simulink model "MIMO_FixedIO"  (R2024a)
settings: Solver=VariableStepAuto  StartTime=0.0  StopTime=10  RelTol=1e-3
undefined symbols (not defined in the file or in its folder): BOOL, DINT, slplc
(part 2 of 5)

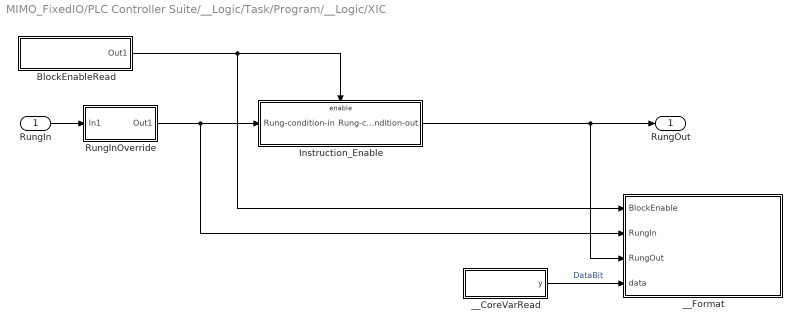
== system MIMO_FixedIO/PLC Controller Suite/__Logic/Task/Program/__Logic/XIC ==
  RungIn : Inport  PortDimensions=1
  BlockEnableRead : Subsystem  DisableCoverage=on  TreatAsAtomicUnit=on  mask{PLCLabelTag=_Block_Enable, PLCBlockType=BlockEnableRead}
      mask prompts: PLCLabelTag "Label Tag:"
      mask init:
      | block = gcb;
      | maskObj = Simulink.Mask.get(block);
      | maskObj.Display = sprintf('disp(''%s'');', PLCLabelTag);
      mask Help: web([docroot '/plccoder/ref/blockenableread' '.html']);
      mask DialogControl PLCBlockTitle Prompt: Block Enable Read
      mask Display: disp('_Block_Enable');
  Instruction_Enable : Subsystem  Priority=12  TreatAsAtomicUnit=on
  RungInOverride : Subsystem  DisableCoverage=on  TreatAsAtomicUnit=on
  __CoreVarRead : Subsystem  Tag=CoreVarReadBlock  DisableCoverage=on  TreatAsAtomicUnit=on  mask{PLCBlockType=CoreVarRead}
      mask init:
      | slplc.callbacks.initCoreVariable(gcb, 'read');
      mask Help: web([docroot '/plccoder/ref/__corevarread' '.html']);
      mask DialogControl PLCBlockTitle Prompt: Core Variable Read
  __Format : MATLAB Function  Tag=PLC_Format_Boolean  Priority=20  DisableCoverage=on  InitFcn=slplc.utils.setBlockAppearance('reset', '%<PLCOperandTag>');  StopFcn=slplc.utils.setBlockAppearance('reset', '%<PLCOperandTag>');  TreatAsAtomicUnit=on
  RungOut : Outport  OutDataTypeStr=BOOL  PortDimensions=1  InitialOutput=false  VectorParamsAs1DForOutWhenUnconnected=off
  wires:
  __CoreVarRead/1(y) -> __Format/4(data)  "DataBit"
  RungInOverride/1(Out1) -> Instruction_Enable/1(Rung-condition-in), __Format/2(RungIn)
  BlockEnableRead/1(Out1) -> Instruction_Enable/Enable, __Format/1(BlockEnable)
  Instruction_Enable/1(Rung-condition-out) -> RungOut/1, __Format/3(RungOut)
  RungIn/1 -> RungInOverride/1(In1)

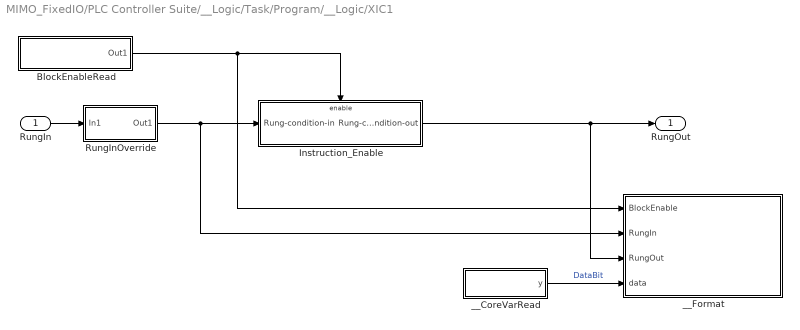
== system MIMO_FixedIO/PLC Controller Suite/__Logic/Task/Program/__Logic/XIC1 ==
  RungIn : Inport  PortDimensions=1
  BlockEnableRead : Subsystem  DisableCoverage=on  TreatAsAtomicUnit=on  mask{PLCLabelTag=_Block_Enable, PLCBlockType=BlockEnableRead}
      mask prompts: PLCLabelTag "Label Tag:"
      mask init:
      | block = gcb;
      | maskObj = Simulink.Mask.get(block);
      | maskObj.Display = sprintf('disp(''%s'');', PLCLabelTag);
      mask Help: web([docroot '/plccoder/ref/blockenableread' '.html']);
      mask DialogControl PLCBlockTitle Prompt: Block Enable Read
      mask Display: disp('_Block_Enable');
  Instruction_Enable : Subsystem  Priority=12  TreatAsAtomicUnit=on
  RungInOverride : Subsystem  DisableCoverage=on  TreatAsAtomicUnit=on
  __CoreVarRead : Subsystem  Tag=CoreVarReadBlock  DisableCoverage=on  TreatAsAtomicUnit=on  mask{PLCBlockType=CoreVarRead}
      mask init:
      | slplc.callbacks.initCoreVariable(gcb, 'read');
      mask Help: web([docroot '/plccoder/ref/__corevarread' '.html']);
      mask DialogControl PLCBlockTitle Prompt: Core Variable Read
  __Format : MATLAB Function  Tag=PLC_Format_Boolean  Priority=20  DisableCoverage=on  InitFcn=slplc.utils.setBlockAppearance('reset', '%<PLCOperandTag>');  StopFcn=slplc.utils.setBlockAppearance('reset', '%<PLCOperandTag>');  TreatAsAtomicUnit=on
  RungOut : Outport  OutDataTypeStr=BOOL  PortDimensions=1  InitialOutput=false  VectorParamsAs1DForOutWhenUnconnected=off
  wires:
  __CoreVarRead/1(y) -> __Format/4(data)  "DataBit"
  RungInOverride/1(Out1) -> Instruction_Enable/1(Rung-condition-in), __Format/2(RungIn)
  BlockEnableRead/1(Out1) -> Instruction_Enable/Enable, __Format/1(BlockEnable)
  Instruction_Enable/1(Rung-condition-out) -> RungOut/1, __Format/3(RungOut)
  RungIn/1 -> RungInOverride/1(In1)

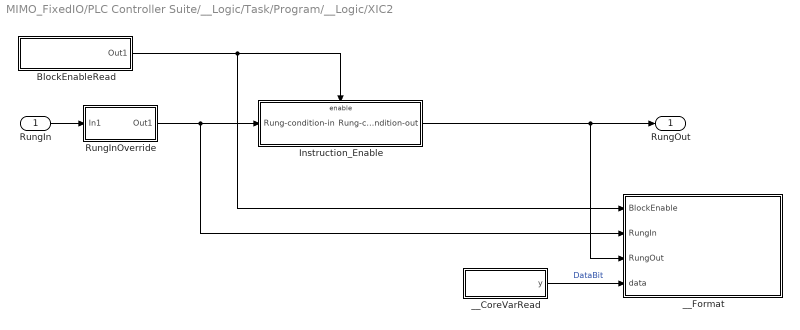
== system MIMO_FixedIO/PLC Controller Suite/__Logic/Task/Program/__Logic/XIC2 ==
  RungIn : Inport  PortDimensions=1
  BlockEnableRead : Subsystem  DisableCoverage=on  TreatAsAtomicUnit=on  mask{PLCLabelTag=_Block_Enable, PLCBlockType=BlockEnableRead}
      mask prompts: PLCLabelTag "Label Tag:"
      mask init:
      | block = gcb;
      | maskObj = Simulink.Mask.get(block);
      | maskObj.Display = sprintf('disp(''%s'');', PLCLabelTag);
      mask Help: web([docroot '/plccoder/ref/blockenableread' '.html']);
      mask DialogControl PLCBlockTitle Prompt: Block Enable Read
      mask Display: disp('_Block_Enable');
  Instruction_Enable : Subsystem  Priority=12  TreatAsAtomicUnit=on
  RungInOverride : Subsystem  DisableCoverage=on  TreatAsAtomicUnit=on
  __CoreVarRead : Subsystem  Tag=CoreVarReadBlock  DisableCoverage=on  TreatAsAtomicUnit=on  mask{PLCBlockType=CoreVarRead}
      mask init:
      | slplc.callbacks.initCoreVariable(gcb, 'read');
      mask Help: web([docroot '/plccoder/ref/__corevarread' '.html']);
      mask DialogControl PLCBlockTitle Prompt: Core Variable Read
  __Format : MATLAB Function  Tag=PLC_Format_Boolean  Priority=20  DisableCoverage=on  InitFcn=slplc.utils.setBlockAppearance('reset', '%<PLCOperandTag>');  StopFcn=slplc.utils.setBlockAppearance('reset', '%<PLCOperandTag>');  TreatAsAtomicUnit=on
  RungOut : Outport  OutDataTypeStr=BOOL  PortDimensions=1  InitialOutput=false  VectorParamsAs1DForOutWhenUnconnected=off
  wires:
  __CoreVarRead/1(y) -> __Format/4(data)  "DataBit"
  RungInOverride/1(Out1) -> Instruction_Enable/1(Rung-condition-in), __Format/2(RungIn)
  BlockEnableRead/1(Out1) -> Instruction_Enable/Enable, __Format/1(BlockEnable)
  Instruction_Enable/1(Rung-condition-out) -> RungOut/1, __Format/3(RungOut)
  RungIn/1 -> RungInOverride/1(In1)

== system MIMO_FixedIO/PLC Controller Suite/__Logic/Task/Program/__Logic/XIC3 ==
  RungIn : Inport  PortDimensions=1
  BlockEnableRead : Subsystem  DisableCoverage=on  TreatAsAtomicUnit=on  mask{PLCLabelTag=_Block_Enable, PLCBlockType=BlockEnableRead}
      mask prompts: PLCLabelTag "Label Tag:"
      mask init:
      | block = gcb;
      | maskObj = Simulink.Mask.get(block);
      | maskObj.Display = sprintf('disp(''%s'');', PLCLabelTag);
      mask Help: web([docroot '/plccoder/ref/blockenableread' '.html']);
      mask DialogControl PLCBlockTitle Prompt: Block Enable Read
      mask Display: disp('_Block_Enable');
  Instruction_Enable : Subsystem  Priority=12  TreatAsAtomicUnit=on
  RungInOverride : Subsystem  DisableCoverage=on  TreatAsAtomicUnit=on
  __CoreVarRead : Subsystem  Tag=CoreVarReadBlock  DisableCoverage=on  TreatAsAtomicUnit=on  mask{PLCBlockType=CoreVarRead}
      mask init:
      | slplc.callbacks.initCoreVariable(gcb, 'read');
      mask Help: web([docroot '/plccoder/ref/__corevarread' '.html']);
      mask DialogControl PLCBlockTitle Prompt: Core Variable Read
  __Format : MATLAB Function  Tag=PLC_Format_Boolean  Priority=20  DisableCoverage=on  InitFcn=slplc.utils.setBlockAppearance('reset', '%<PLCOperandTag>');  StopFcn=slplc.utils.setBlockAppearance('reset', '%<PLCOperandTag>');  TreatAsAtomicUnit=on
  RungOut : Outport  OutDataTypeStr=BOOL  PortDimensions=1  InitialOutput=false  VectorParamsAs1DForOutWhenUnconnected=off
  wires:
  __CoreVarRead/1(y) -> __Format/4(data)  "DataBit"
  RungInOverride/1(Out1) -> Instruction_Enable/1(Rung-condition-in), __Format/2(RungIn)
  BlockEnableRead/1(Out1) -> Instruction_Enable/Enable, __Format/1(BlockEnable)
  Instruction_Enable/1(Rung-condition-out) -> RungOut/1, __Format/3(RungOut)
  RungIn/1 -> RungInOverride/1(In1)

== system MIMO_FixedIO/PLC Controller Suite/__Logic/Task/Program/__Logic/XIC4 ==
  RungIn : Inport  PortDimensions=1
  BlockEnableRead : Subsystem  DisableCoverage=on  TreatAsAtomicUnit=on  mask{PLCLabelTag=_Block_Enable, PLCBlockType=BlockEnableRead}
      mask prompts: PLCLabelTag "Label Tag:"
      mask init:
      | block = gcb;
      | maskObj = Simulink.Mask.get(block);
      | maskObj.Display = sprintf('disp(''%s'');', PLCLabelTag);
      mask Help: web([docroot '/plccoder/ref/blockenableread' '.html']);
      mask DialogControl PLCBlockTitle Prompt: Block Enable Read
      mask Display: disp('_Block_Enable');
  Instruction_Enable : Subsystem  Priority=12  TreatAsAtomicUnit=on
  RungInOverride : Subsystem  DisableCoverage=on  TreatAsAtomicUnit=on
  __CoreVarRead : Subsystem  Tag=CoreVarReadBlock  DisableCoverage=on  TreatAsAtomicUnit=on  mask{PLCBlockType=CoreVarRead}
      mask init:
      | slplc.callbacks.initCoreVariable(gcb, 'read');
      mask Help: web([docroot '/plccoder/ref/__corevarread' '.html']);
      mask DialogControl PLCBlockTitle Prompt: Core Variable Read
  __Format : MATLAB Function  Tag=PLC_Format_Boolean  Priority=20  DisableCoverage=on  InitFcn=slplc.utils.setBlockAppearance('reset', '%<PLCOperandTag>');  StopFcn=slplc.utils.setBlockAppearance('reset', '%<PLCOperandTag>');  TreatAsAtomicUnit=on
  RungOut : Outport  OutDataTypeStr=BOOL  PortDimensions=1  InitialOutput=false  VectorParamsAs1DForOutWhenUnconnected=off
  wires:
  __CoreVarRead/1(y) -> __Format/4(data)  "DataBit"
  RungInOverride/1(Out1) -> Instruction_Enable/1(Rung-condition-in), __Format/2(RungIn)
  BlockEnableRead/1(Out1) -> Instruction_Enable/Enable, __Format/1(BlockEnable)
  Instruction_Enable/1(Rung-condition-out) -> RungOut/1, __Format/3(RungOut)
  RungIn/1 -> RungInOverride/1(In1)

== system MIMO_FixedIO/PLC Controller Suite/__Logic/Task/Program/__Logic/XIC5 ==
  RungIn : Inport  PortDimensions=1
  BlockEnableRead : Subsystem  DisableCoverage=on  TreatAsAtomicUnit=on  mask{PLCLabelTag=_Block_Enable, PLCBlockType=BlockEnableRead}
      mask prompts: PLCLabelTag "Label Tag:"
      mask init:
      | block = gcb;
      | maskObj = Simulink.Mask.get(block);
      | maskObj.Display = sprintf('disp(''%s'');', PLCLabelTag);
      mask Help: web([docroot '/plccoder/ref/blockenableread' '.html']);
      mask DialogControl PLCBlockTitle Prompt: Block Enable Read
      mask Display: disp('_Block_Enable');
  Instruction_Enable : Subsystem  Priority=12  TreatAsAtomicUnit=on
  RungInOverride : Subsystem  DisableCoverage=on  TreatAsAtomicUnit=on
  __CoreVarRead : Subsystem  Tag=CoreVarReadBlock  DisableCoverage=on  TreatAsAtomicUnit=on  mask{PLCBlockType=CoreVarRead}
      mask init:
      | slplc.callbacks.initCoreVariable(gcb, 'read');
      mask Help: web([docroot '/plccoder/ref/__corevarread' '.html']);
      mask DialogControl PLCBlockTitle Prompt: Core Variable Read
  __Format : MATLAB Function  Tag=PLC_Format_Boolean  Priority=20  DisableCoverage=on  InitFcn=slplc.utils.setBlockAppearance('reset', '%<PLCOperandTag>');  StopFcn=slplc.utils.setBlockAppearance('reset', '%<PLCOperandTag>');  TreatAsAtomicUnit=on
  RungOut : Outport  OutDataTypeStr=BOOL  PortDimensions=1  InitialOutput=false  VectorParamsAs1DForOutWhenUnconnected=off
  wires:
  __CoreVarRead/1(y) -> __Format/4(data)  "DataBit"
  RungInOverride/1(Out1) -> Instruction_Enable/1(Rung-condition-in), __Format/2(RungIn)
  BlockEnableRead/1(Out1) -> Instruction_Enable/Enable, __Format/1(BlockEnable)
  Instruction_Enable/1(Rung-condition-out) -> RungOut/1, __Format/3(RungOut)
  RungIn/1 -> RungInOverride/1(In1)

== system MIMO_FixedIO/PLC Controller Suite/__Logic/Task/Program/__Logic/XIC6 ==
  RungIn : Inport  PortDimensions=1
  BlockEnableRead : Subsystem  DisableCoverage=on  TreatAsAtomicUnit=on  mask{PLCLabelTag=_Block_Enable, PLCBlockType=BlockEnableRead}
      mask prompts: PLCLabelTag "Label Tag:"
      mask init:
      | block = gcb;
      | maskObj = Simulink.Mask.get(block);
      | maskObj.Display = sprintf('disp(''%s'');', PLCLabelTag);
      mask Help: web([docroot '/plccoder/ref/blockenableread' '.html']);
      mask DialogControl PLCBlockTitle Prompt: Block Enable Read
      mask Display: disp('_Block_Enable');
  Instruction_Enable : Subsystem  Priority=12  TreatAsAtomicUnit=on
  RungInOverride : Subsystem  DisableCoverage=on  TreatAsAtomicUnit=on
  __CoreVarRead : Subsystem  Tag=CoreVarReadBlock  DisableCoverage=on  TreatAsAtomicUnit=on  mask{PLCBlockType=CoreVarRead}
      mask init:
      | slplc.callbacks.initCoreVariable(gcb, 'read');
      mask Help: web([docroot '/plccoder/ref/__corevarread' '.html']);
      mask DialogControl PLCBlockTitle Prompt: Core Variable Read
  __Format : MATLAB Function  Tag=PLC_Format_Boolean  Priority=20  DisableCoverage=on  InitFcn=slplc.utils.setBlockAppearance('reset', '%<PLCOperandTag>');  StopFcn=slplc.utils.setBlockAppearance('reset', '%<PLCOperandTag>');  TreatAsAtomicUnit=on
  RungOut : Outport  OutDataTypeStr=BOOL  PortDimensions=1  InitialOutput=false  VectorParamsAs1DForOutWhenUnconnected=off
  wires:
  __CoreVarRead/1(y) -> __Format/4(data)  "DataBit"
  RungInOverride/1(Out1) -> Instruction_Enable/1(Rung-condition-in), __Format/2(RungIn)
  BlockEnableRead/1(Out1) -> Instruction_Enable/Enable, __Format/1(BlockEnable)
  Instruction_Enable/1(Rung-condition-out) -> RungOut/1, __Format/3(RungOut)
  RungIn/1 -> RungInOverride/1(In1)

== system MIMO_FixedIO/PLC Controller Suite/__Logic/Task/Program/__Logic/XIC8 ==
  RungIn : Inport  PortDimensions=1
  BlockEnableRead : Subsystem  DisableCoverage=on  TreatAsAtomicUnit=on  mask{PLCLabelTag=_Block_Enable, PLCBlockType=BlockEnableRead}
      mask prompts: PLCLabelTag "Label Tag:"
      mask init:
      | block = gcb;
      | maskObj = Simulink.Mask.get(block);
      | maskObj.Display = sprintf('disp(''%s'');', PLCLabelTag);
      mask Help: web([docroot '/plccoder/ref/blockenableread' '.html']);
      mask DialogControl PLCBlockTitle Prompt: Block Enable Read
      mask Display: disp('_Block_Enable');
  Instruction_Enable : Subsystem  Priority=12  TreatAsAtomicUnit=on
  RungInOverride : Subsystem  DisableCoverage=on  TreatAsAtomicUnit=on
  __CoreVarRead : Subsystem  Tag=CoreVarReadBlock  DisableCoverage=on  TreatAsAtomicUnit=on  mask{PLCBlockType=CoreVarRead}
      mask init:
      | slplc.callbacks.initCoreVariable(gcb, 'read');
      mask Help: web([docroot '/plccoder/ref/__corevarread' '.html']);
      mask DialogControl PLCBlockTitle Prompt: Core Variable Read
  __Format : MATLAB Function  Tag=PLC_Format_Boolean  Priority=20  DisableCoverage=on  InitFcn=slplc.utils.setBlockAppearance('reset', '%<PLCOperandTag>');  StopFcn=slplc.utils.setBlockAppearance('reset', '%<PLCOperandTag>');  TreatAsAtomicUnit=on
  RungOut : Outport  OutDataTypeStr=BOOL  PortDimensions=1  InitialOutput=false  VectorParamsAs1DForOutWhenUnconnected=off
  wires:
  __CoreVarRead/1(y) -> __Format/4(data)  "DataBit"
  RungInOverride/1(Out1) -> Instruction_Enable/1(Rung-condition-in), __Format/2(RungIn)
  BlockEnableRead/1(Out1) -> Instruction_Enable/Enable, __Format/1(BlockEnable)
  Instruction_Enable/1(Rung-condition-out) -> RungOut/1, __Format/3(RungOut)
  RungIn/1 -> RungInOverride/1(In1)

== system MIMO_FixedIO/PLC Controller Suite/__Logic/Task/Program/__Logic/XIC9 ==
  RungIn : Inport  PortDimensions=1
  BlockEnableRead : Subsystem  DisableCoverage=on  TreatAsAtomicUnit=on  mask{PLCLabelTag=_Block_Enable, PLCBlockType=BlockEnableRead}
      mask prompts: PLCLabelTag "Label Tag:"
      mask init:
      | block = gcb;
      | maskObj = Simulink.Mask.get(block);
      | maskObj.Display = sprintf('disp(''%s'');', PLCLabelTag);
      mask Help: web([docroot '/plccoder/ref/blockenableread' '.html']);
      mask DialogControl PLCBlockTitle Prompt: Block Enable Read
      mask Display: disp('_Block_Enable');
  Instruction_Enable : Subsystem  Priority=12  TreatAsAtomicUnit=on
  RungInOverride : Subsystem  DisableCoverage=on  TreatAsAtomicUnit=on
  __CoreVarRead : Subsystem  Tag=CoreVarReadBlock  DisableCoverage=on  TreatAsAtomicUnit=on  mask{PLCBlockType=CoreVarRead}
      mask init:
      | slplc.callbacks.initCoreVariable(gcb, 'read');
      mask Help: web([docroot '/plccoder/ref/__corevarread' '.html']);
      mask DialogControl PLCBlockTitle Prompt: Core Variable Read
  __Format : MATLAB Function  Tag=PLC_Format_Boolean  Priority=20  DisableCoverage=on  InitFcn=slplc.utils.setBlockAppearance('reset', '%<PLCOperandTag>');  StopFcn=slplc.utils.setBlockAppearance('reset', '%<PLCOperandTag>');  TreatAsAtomicUnit=on
  RungOut : Outport  OutDataTypeStr=BOOL  PortDimensions=1  InitialOutput=false  VectorParamsAs1DForOutWhenUnconnected=off
  wires:
  __CoreVarRead/1(y) -> __Format/4(data)  "DataBit"
  RungInOverride/1(Out1) -> Instruction_Enable/1(Rung-condition-in), __Format/2(RungIn)
  BlockEnableRead/1(Out1) -> Instruction_Enable/Enable, __Format/1(BlockEnable)
  Instruction_Enable/1(Rung-condition-out) -> RungOut/1, __Format/3(RungOut)
  RungIn/1 -> RungInOverride/1(In1)

== system MIMO_FixedIO/PLC Controller Suite/__Logic/Task/Program/__Logic/XIO ==
  RungIn : Inport  PortDimensions=1
  BlockEnableRead : Subsystem  DisableCoverage=on  TreatAsAtomicUnit=on  mask{PLCLabelTag=_Block_Enable, PLCBlockType=BlockEnableRead}
      mask prompts: PLCLabelTag "Label Tag:"
      mask init:
      | block = gcb;
      | maskObj = Simulink.Mask.get(block);
      | maskObj.Display = sprintf('disp(''%s'');', PLCLabelTag);
      mask Help: web([docroot '/plccoder/ref/blockenableread' '.html']);
      mask DialogControl PLCBlockTitle Prompt: Block Enable Read
      mask Display: disp('_Block_Enable');
  Instruction_Enable : Subsystem  Priority=12  TreatAsAtomicUnit=on
  RungInOverride : Subsystem  DisableCoverage=on  TreatAsAtomicUnit=on
  __CoreVarRead : Subsystem  Tag=CoreVarReadBlock  DisableCoverage=on  TreatAsAtomicUnit=on  mask{PLCBlockType=CoreVarRead}
      mask init:
      | slplc.callbacks.initCoreVariable(gcb, 'read');
      mask Help: web([docroot '/plccoder/ref/__corevarread' '.html']);
      mask DialogControl PLCBlockTitle Prompt: Core Variable Read
  __Format : MATLAB Function  Tag=PLC_Format_Boolean  Priority=20  DisableCoverage=on  InitFcn=slplc.utils.setBlockAppearance('reset', '%<PLCOperandTag>');  StopFcn=slplc.utils.setBlockAppearance('reset', '%<PLCOperandTag>');  TreatAsAtomicUnit=on
  RungOut : Outport  OutDataTypeStr=BOOL  PortDimensions=1  InitialOutput=false  VectorParamsAs1DForOutWhenUnconnected=off
  wires:
  BlockEnableRead/1(Out1) -> Instruction_Enable/Enable, __Format/1(BlockEnable)
  RungIn/1 -> RungInOverride/1(In1)
  Instruction_Enable/1(Rung-condition-out) -> __Format/3(RungOut), RungOut/1
  RungInOverride/1(Out1) -> Instruction_Enable/1(Rung-condition-in), __Format/2(RungIn)
  __CoreVarRead/1(y) -> __Format/4(data)  "DataBit"

== system MIMO_FixedIO/PLC Controller Suite/__Logic/Task/Program/__Logic/XIO1 ==
  RungIn : Inport  PortDimensions=1
  BlockEnableRead : Subsystem  DisableCoverage=on  TreatAsAtomicUnit=on  mask{PLCLabelTag=_Block_Enable, PLCBlockType=BlockEnableRead}
      mask prompts: PLCLabelTag "Label Tag:"
      mask init:
      | block = gcb;
      | maskObj = Simulink.Mask.get(block);
      | maskObj.Display = sprintf('disp(''%s'');', PLCLabelTag);
      mask Help: web([docroot '/plccoder/ref/blockenableread' '.html']);
      mask DialogControl PLCBlockTitle Prompt: Block Enable Read
      mask Display: disp('_Block_Enable');
  Instruction_Enable : Subsystem  Priority=12  TreatAsAtomicUnit=on
  RungInOverride : Subsystem  DisableCoverage=on  TreatAsAtomicUnit=on
  __CoreVarRead : Subsystem  Tag=CoreVarReadBlock  DisableCoverage=on  TreatAsAtomicUnit=on  mask{PLCBlockType=CoreVarRead}
      mask init:
      | slplc.callbacks.initCoreVariable(gcb, 'read');
      mask Help: web([docroot '/plccoder/ref/__corevarread' '.html']);
      mask DialogControl PLCBlockTitle Prompt: Core Variable Read
  __Format : MATLAB Function  Tag=PLC_Format_Boolean  Priority=20  DisableCoverage=on  InitFcn=slplc.utils.setBlockAppearance('reset', '%<PLCOperandTag>');  StopFcn=slplc.utils.setBlockAppearance('reset', '%<PLCOperandTag>');  TreatAsAtomicUnit=on
  RungOut : Outport  OutDataTypeStr=BOOL  PortDimensions=1  InitialOutput=false  VectorParamsAs1DForOutWhenUnconnected=off
  wires:
  BlockEnableRead/1(Out1) -> Instruction_Enable/Enable, __Format/1(BlockEnable)
  RungIn/1 -> RungInOverride/1(In1)
  Instruction_Enable/1(Rung-condition-out) -> __Format/3(RungOut), RungOut/1
  RungInOverride/1(Out1) -> Instruction_Enable/1(Rung-condition-in), __Format/2(RungIn)
  __CoreVarRead/1(y) -> __Format/4(data)  "DataBit"

== system MIMO_FixedIO/PLC Controller Suite/__Logic/Task/Program/__Logic/XIO2 ==
  RungIn : Inport  PortDimensions=1
  BlockEnableRead : Subsystem  DisableCoverage=on  TreatAsAtomicUnit=on  mask{PLCLabelTag=_Block_Enable, PLCBlockType=BlockEnableRead}
      mask prompts: PLCLabelTag "Label Tag:"
      mask init:
      | block = gcb;
      | maskObj = Simulink.Mask.get(block);
      | maskObj.Display = sprintf('disp(''%s'');', PLCLabelTag);
      mask Help: web([docroot '/plccoder/ref/blockenableread' '.html']);
      mask DialogControl PLCBlockTitle Prompt: Block Enable Read
      mask Display: disp('_Block_Enable');
  Instruction_Enable : Subsystem  Priority=12  TreatAsAtomicUnit=on
  RungInOverride : Subsystem  DisableCoverage=on  TreatAsAtomicUnit=on
  __CoreVarRead : Subsystem  Tag=CoreVarReadBlock  DisableCoverage=on  TreatAsAtomicUnit=on  mask{PLCBlockType=CoreVarRead}
      mask init:
      | slplc.callbacks.initCoreVariable(gcb, 'read');
      mask Help: web([docroot '/plccoder/ref/__corevarread' '.html']);
      mask DialogControl PLCBlockTitle Prompt: Core Variable Read
  __Format : MATLAB Function  Tag=PLC_Format_Boolean  Priority=20  DisableCoverage=on  InitFcn=slplc.utils.setBlockAppearance('reset', '%<PLCOperandTag>');  StopFcn=slplc.utils.setBlockAppearance('reset', '%<PLCOperandTag>');  TreatAsAtomicUnit=on
  RungOut : Outport  OutDataTypeStr=BOOL  PortDimensions=1  InitialOutput=false  VectorParamsAs1DForOutWhenUnconnected=off
  wires:
  BlockEnableRead/1(Out1) -> Instruction_Enable/Enable, __Format/1(BlockEnable)
  RungIn/1 -> RungInOverride/1(In1)
  Instruction_Enable/1(Rung-condition-out) -> __Format/3(RungOut), RungOut/1
  RungInOverride/1(Out1) -> Instruction_Enable/1(Rung-condition-in), __Format/2(RungIn)
  __CoreVarRead/1(y) -> __Format/4(data)  "DataBit"

== system MIMO_FixedIO/PLC Controller Suite/__Logic/Task/Program/__Logic/XIO3 ==
  RungIn : Inport  PortDimensions=1
  BlockEnableRead : Subsystem  DisableCoverage=on  TreatAsAtomicUnit=on  mask{PLCLabelTag=_Block_Enable, PLCBlockType=BlockEnableRead}
      mask prompts: PLCLabelTag "Label Tag:"
      mask init:
      | block = gcb;
      | maskObj = Simulink.Mask.get(block);
      | maskObj.Display = sprintf('disp(''%s'');', PLCLabelTag);
      mask Help: web([docroot '/plccoder/ref/blockenableread' '.html']);
      mask DialogControl PLCBlockTitle Prompt: Block Enable Read
      mask Display: disp('_Block_Enable');
  Instruction_Enable : Subsystem  Priority=12  TreatAsAtomicUnit=on
  RungInOverride : Subsystem  DisableCoverage=on  TreatAsAtomicUnit=on
  __CoreVarRead : Subsystem  Tag=CoreVarReadBlock  DisableCoverage=on  TreatAsAtomicUnit=on  mask{PLCBlockType=CoreVarRead}
      mask init:
      | slplc.callbacks.initCoreVariable(gcb, 'read');
      mask Help: web([docroot '/plccoder/ref/__corevarread' '.html']);
      mask DialogControl PLCBlockTitle Prompt: Core Variable Read
  __Format : MATLAB Function  Tag=PLC_Format_Boolean  Priority=20  DisableCoverage=on  InitFcn=slplc.utils.setBlockAppearance('reset', '%<PLCOperandTag>');  StopFcn=slplc.utils.setBlockAppearance('reset', '%<PLCOperandTag>');  TreatAsAtomicUnit=on
  RungOut : Outport  OutDataTypeStr=BOOL  PortDimensions=1  InitialOutput=false  VectorParamsAs1DForOutWhenUnconnected=off
  wires:
  BlockEnableRead/1(Out1) -> Instruction_Enable/Enable, __Format/1(BlockEnable)
  RungIn/1 -> RungInOverride/1(In1)
  Instruction_Enable/1(Rung-condition-out) -> __Format/3(RungOut), RungOut/1
  RungInOverride/1(Out1) -> Instruction_Enable/1(Rung-condition-in), __Format/2(RungIn)
  __CoreVarRead/1(y) -> __Format/4(data)  "DataBit"

== system MIMO_FixedIO/PLC Controller Suite/__Logic/Task/Program/__Logic/XIO4 ==
  RungIn : Inport  PortDimensions=1
  BlockEnableRead : Subsystem  DisableCoverage=on  TreatAsAtomicUnit=on  mask{PLCLabelTag=_Block_Enable, PLCBlockType=BlockEnableRead}
      mask prompts: PLCLabelTag "Label Tag:"
      mask init:
      | block = gcb;
      | maskObj = Simulink.Mask.get(block);
      | maskObj.Display = sprintf('disp(''%s'');', PLCLabelTag);
      mask Help: web([docroot '/plccoder/ref/blockenableread' '.html']);
      mask DialogControl PLCBlockTitle Prompt: Block Enable Read
      mask Display: disp('_Block_Enable');
  Instruction_Enable : Subsystem  Priority=12  TreatAsAtomicUnit=on
  RungInOverride : Subsystem  DisableCoverage=on  TreatAsAtomicUnit=on
  __CoreVarRead : Subsystem  Tag=CoreVarReadBlock  DisableCoverage=on  TreatAsAtomicUnit=on  mask{PLCBlockType=CoreVarRead}
      mask init:
      | slplc.callbacks.initCoreVariable(gcb, 'read');
      mask Help: web([docroot '/plccoder/ref/__corevarread' '.html']);
      mask DialogControl PLCBlockTitle Prompt: Core Variable Read
  __Format : MATLAB Function  Tag=PLC_Format_Boolean  Priority=20  DisableCoverage=on  InitFcn=slplc.utils.setBlockAppearance('reset', '%<PLCOperandTag>');  StopFcn=slplc.utils.setBlockAppearance('reset', '%<PLCOperandTag>');  TreatAsAtomicUnit=on
  RungOut : Outport  OutDataTypeStr=BOOL  PortDimensions=1  InitialOutput=false  VectorParamsAs1DForOutWhenUnconnected=off
  wires:
  BlockEnableRead/1(Out1) -> Instruction_Enable/Enable, __Format/1(BlockEnable)
  RungIn/1 -> RungInOverride/1(In1)
  Instruction_Enable/1(Rung-condition-out) -> __Format/3(RungOut), RungOut/1
  RungInOverride/1(Out1) -> Instruction_Enable/1(Rung-condition-in), __Format/2(RungIn)
  __CoreVarRead/1(y) -> __Format/4(data)  "DataBit"

== system MIMO_FixedIO/PLC Controller Suite/__Logic/Task/Program/__Logic/XIO5 ==
  RungIn : Inport  PortDimensions=1
  BlockEnableRead : Subsystem  DisableCoverage=on  TreatAsAtomicUnit=on  mask{PLCLabelTag=_Block_Enable, PLCBlockType=BlockEnableRead}
      mask prompts: PLCLabelTag "Label Tag:"
      mask init:
      | block = gcb;
      | maskObj = Simulink.Mask.get(block);
      | maskObj.Display = sprintf('disp(''%s'');', PLCLabelTag);
      mask Help: web([docroot '/plccoder/ref/blockenableread' '.html']);
      mask DialogControl PLCBlockTitle Prompt: Block Enable Read
      mask Display: disp('_Block_Enable');
  Instruction_Enable : Subsystem  Priority=12  TreatAsAtomicUnit=on
  RungInOverride : Subsystem  DisableCoverage=on  TreatAsAtomicUnit=on
  __CoreVarRead : Subsystem  Tag=CoreVarReadBlock  DisableCoverage=on  TreatAsAtomicUnit=on  mask{PLCBlockType=CoreVarRead}
      mask init:
      | slplc.callbacks.initCoreVariable(gcb, 'read');
      mask Help: web([docroot '/plccoder/ref/__corevarread' '.html']);
      mask DialogControl PLCBlockTitle Prompt: Core Variable Read
  __Format : MATLAB Function  Tag=PLC_Format_Boolean  Priority=20  DisableCoverage=on  InitFcn=slplc.utils.setBlockAppearance('reset', '%<PLCOperandTag>');  StopFcn=slplc.utils.setBlockAppearance('reset', '%<PLCOperandTag>');  TreatAsAtomicUnit=on
  RungOut : Outport  OutDataTypeStr=BOOL  PortDimensions=1  InitialOutput=false  VectorParamsAs1DForOutWhenUnconnected=off
  wires:
  BlockEnableRead/1(Out1) -> Instruction_Enable/Enable, __Format/1(BlockEnable)
  RungIn/1 -> RungInOverride/1(In1)
  Instruction_Enable/1(Rung-condition-out) -> __Format/3(RungOut), RungOut/1
  RungInOverride/1(Out1) -> Instruction_Enable/1(Rung-condition-in), __Format/2(RungIn)
  __CoreVarRead/1(y) -> __Format/4(data)  "DataBit"

== system MIMO_FixedIO/PLC Controller Suite/__Logic/Task/Program/__Logic/XIO6 ==
  RungIn : Inport  PortDimensions=1
  BlockEnableRead : Subsystem  DisableCoverage=on  TreatAsAtomicUnit=on  mask{PLCLabelTag=_Block_Enable, PLCBlockType=BlockEnableRead}
      mask prompts: PLCLabelTag "Label Tag:"
      mask init:
      | block = gcb;
      | maskObj = Simulink.Mask.get(block);
      | maskObj.Display = sprintf('disp(''%s'');', PLCLabelTag);
      mask Help: web([docroot '/plccoder/ref/blockenableread' '.html']);
      mask DialogControl PLCBlockTitle Prompt: Block Enable Read
      mask Display: disp('_Block_Enable');
  Instruction_Enable : Subsystem  Priority=12  TreatAsAtomicUnit=on
  RungInOverride : Subsystem  DisableCoverage=on  TreatAsAtomicUnit=on
  __CoreVarRead : Subsystem  Tag=CoreVarReadBlock  DisableCoverage=on  TreatAsAtomicUnit=on  mask{PLCBlockType=CoreVarRead}
      mask init:
      | slplc.callbacks.initCoreVariable(gcb, 'read');
      mask Help: web([docroot '/plccoder/ref/__corevarread' '.html']);
      mask DialogControl PLCBlockTitle Prompt: Core Variable Read
  __Format : MATLAB Function  Tag=PLC_Format_Boolean  Priority=20  DisableCoverage=on  InitFcn=slplc.utils.setBlockAppearance('reset', '%<PLCOperandTag>');  StopFcn=slplc.utils.setBlockAppearance('reset', '%<PLCOperandTag>');  TreatAsAtomicUnit=on
  RungOut : Outport  OutDataTypeStr=BOOL  PortDimensions=1  InitialOutput=false  VectorParamsAs1DForOutWhenUnconnected=off
  wires:
  BlockEnableRead/1(Out1) -> Instruction_Enable/Enable, __Format/1(BlockEnable)
  RungIn/1 -> RungInOverride/1(In1)
  Instruction_Enable/1(Rung-condition-out) -> __Format/3(RungOut), RungOut/1
  RungInOverride/1(Out1) -> Instruction_Enable/1(Rung-condition-in), __Format/2(RungIn)
  __CoreVarRead/1(y) -> __Format/4(data)  "DataBit"

== system MIMO_FixedIO/PLC Controller Suite/__Logic/Task/Program/__Logic/Junction/BlockEnableRead ==
  __CoreLabelRead : Subsystem  Tag=CoreVarReadBlock  DisableCoverage=on  TreatAsAtomicUnit=on  mask{PLCBlockType=CoreLabelRead}
      mask init:
      | slplc.callbacks.initRoutineLabelRead(gcb);
      mask Help: web([docroot '/plccoder/ref/__corelabelread' '.html']);
      mask DialogControl PLCBlockTitle Prompt: Core Label Read
  Out1 : Outport  VectorParamsAs1DForOutWhenUnconnected=off
  wires:
  __CoreLabelRead/1(Out1) -> Out1/1

== system MIMO_FixedIO/PLC Controller Suite/__Logic/Task/Program/__Logic/Junction/__Enable ==
  RungIn1 : Inport
  RungIn2 : Inport  Port=2
  Enable : EnablePort
  Logical Operator : Logic  Operator=OR  AllPortsSameDT=off  OutDataTypeStr=BOOL
  RungOut : Outport  VectorParamsAs1DForOutWhenUnconnected=off
  wires:
  RungIn2/1 -> Logical Operator/2
  Logical Operator/1 -> RungOut/1
  RungIn1/1 -> Logical Operator/1

== system MIMO_FixedIO/PLC Controller Suite/__Logic/Task/Program/__Logic/Junction1/BlockEnableRead ==
  __CoreLabelRead : Subsystem  Tag=CoreVarReadBlock  DisableCoverage=on  TreatAsAtomicUnit=on  mask{PLCBlockType=CoreLabelRead}
      mask init:
      | slplc.callbacks.initRoutineLabelRead(gcb);
      mask Help: web([docroot '/plccoder/ref/__corelabelread' '.html']);
      mask DialogControl PLCBlockTitle Prompt: Core Label Read
  Out1 : Outport  VectorParamsAs1DForOutWhenUnconnected=off
  wires:
  __CoreLabelRead/1(Out1) -> Out1/1

== system MIMO_FixedIO/PLC Controller Suite/__Logic/Task/Program/__Logic/Junction1/__Enable ==
  RungIn1 : Inport
  RungIn2 : Inport  Port=2
  Enable : EnablePort
  Logical Operator : Logic  Operator=OR  AllPortsSameDT=off  OutDataTypeStr=BOOL
  RungOut : Outport  VectorParamsAs1DForOutWhenUnconnected=off
  wires:
  RungIn2/1 -> Logical Operator/2
  Logical Operator/1 -> RungOut/1
  RungIn1/1 -> Logical Operator/1

== system MIMO_FixedIO/PLC Controller Suite/__Logic/Task/Program/__Logic/Junction2/BlockEnableRead ==
  __CoreLabelRead : Subsystem  Tag=CoreVarReadBlock  DisableCoverage=on  TreatAsAtomicUnit=on  mask{PLCBlockType=CoreLabelRead}
      mask init:
      | slplc.callbacks.initRoutineLabelRead(gcb);
      mask Help: web([docroot '/plccoder/ref/__corelabelread' '.html']);
      mask DialogControl PLCBlockTitle Prompt: Core Label Read
  Out1 : Outport  VectorParamsAs1DForOutWhenUnconnected=off
  wires:
  __CoreLabelRead/1(Out1) -> Out1/1

== system MIMO_FixedIO/PLC Controller Suite/__Logic/Task/Program/__Logic/Junction2/__Enable ==
  RungIn1 : Inport
  RungIn2 : Inport  Port=2
  Enable : EnablePort
  Logical Operator : Logic  Operator=OR  AllPortsSameDT=off  OutDataTypeStr=BOOL
  RungOut : Outport  VectorParamsAs1DForOutWhenUnconnected=off
  wires:
  RungIn2/1 -> Logical Operator/2
  Logical Operator/1 -> RungOut/1
  RungIn1/1 -> Logical Operator/1

== system MIMO_FixedIO/PLC Controller Suite/__Logic/Task/Program/__Logic/OTE/BlockEnableRead ==
  __CoreLabelRead : Subsystem  Tag=CoreVarReadBlock  DisableCoverage=on  TreatAsAtomicUnit=on  mask{PLCBlockType=CoreLabelRead}
      mask init:
      | slplc.callbacks.initRoutineLabelRead(gcb);
      mask Help: web([docroot '/plccoder/ref/__corelabelread' '.html']);
      mask DialogControl PLCBlockTitle Prompt: Core Label Read
  Out1 : Outport  VectorParamsAs1DForOutWhenUnconnected=off
  wires:
  __CoreLabelRead/1(Out1) -> Out1/1

== system MIMO_FixedIO/PLC Controller Suite/__Logic/Task/Program/__Logic/OTE/Instruction_Enable ==
  Rung-condition-in : Inport  OutDataTypeStr=BOOL
  Enable : EnablePort
  Initialize Function : Subsystem  TreatAsAtomicUnit=on
  NOT : Logic  Operator=NOT  IconShape=distinctive  AllPortsSameDT=off  OutDataTypeStr=boolean
  Rung-condition is false : Subsystem  Priority=12  DisableCoverage=on
  Rung-condition-in is true : Subsystem  Priority=12  DisableCoverage=on
  wires:
  NOT/1 -> Rung-condition is false/Enable
  Rung-condition-in/1 -> Rung-condition-in is true/Enable, NOT/1  "Rung-condition-in"

== system MIMO_FixedIO/PLC Controller Suite/__Logic/Task/Program/__Logic/OTE/RungInOverride ==
  In1 : Inport
  AND : Logic  AllPortsSameDT=off  OutDataTypeStr=boolean
  ForceRungInFalseRead : Subsystem  DisableCoverage=on  TreatAsAtomicUnit=on  mask{PLCLabelTag=_Force_RungIn_False, PLCBlockType=ForceRungInFalseRead}
      mask prompts: PLCLabelTag "Label Tag:"
      mask init:
      | block = gcb;
      | maskObj = Simulink.Mask.get(block);
      | maskObj.Display = sprintf('disp(''%s'');', PLCLabelTag);
      mask Help: web([docroot '/plccoder/ref/forcerunginfalseread' '.html']);
      mask DialogControl PLCBlockTitle Prompt: Force Rung-In False Read
      mask Display: disp('_Force_RungIn_False');
  NOT : Logic  Operator=NOT  IconShape=distinctive  AllPortsSameDT=off  OutDataTypeStr=boolean
  Out1 : Outport  VectorParamsAs1DForOutWhenUnconnected=off
  wires:
  AND/1 -> Out1/1
  In1/1 -> AND/2
  ForceRungInFalseRead/1(Out1) -> NOT/1
  NOT/1 -> AND/1

== system MIMO_FixedIO/PLC Controller Suite/__Logic/Task/Program/__Logic/OTE/__CoreVarRead ==
  DataRead : DataStoreRead  DataStoreName=xxx_PLC_VAR_State0  IndexOptions=Index vector (dialog)  Indices=1  OutputSizes=1
  y : Outport  VectorParamsAs1DForOutWhenUnconnected=off
  wires:
  DataRead/1 -> y/1

== system MIMO_FixedIO/PLC Controller Suite/__Logic/Task/Program/__Logic/OTE1/BlockEnableRead ==
  __CoreLabelRead : Subsystem  Tag=CoreVarReadBlock  DisableCoverage=on  TreatAsAtomicUnit=on  mask{PLCBlockType=CoreLabelRead}
      mask init:
      | slplc.callbacks.initRoutineLabelRead(gcb);
      mask Help: web([docroot '/plccoder/ref/__corelabelread' '.html']);
      mask DialogControl PLCBlockTitle Prompt: Core Label Read
  Out1 : Outport  VectorParamsAs1DForOutWhenUnconnected=off
  wires:
  __CoreLabelRead/1(Out1) -> Out1/1

== system MIMO_FixedIO/PLC Controller Suite/__Logic/Task/Program/__Logic/OTE1/Instruction_Enable ==
  Rung-condition-in : Inport  OutDataTypeStr=BOOL
  Enable : EnablePort
  Initialize Function : Subsystem  TreatAsAtomicUnit=on
  NOT : Logic  Operator=NOT  IconShape=distinctive  AllPortsSameDT=off  OutDataTypeStr=boolean
  Rung-condition is false : Subsystem  Priority=12  DisableCoverage=on
  Rung-condition-in is true : Subsystem  Priority=12  DisableCoverage=on
  wires:
  NOT/1 -> Rung-condition is false/Enable
  Rung-condition-in/1 -> Rung-condition-in is true/Enable, NOT/1  "Rung-condition-in"

== system MIMO_FixedIO/PLC Controller Suite/__Logic/Task/Program/__Logic/OTE1/RungInOverride ==
  In1 : Inport
  AND : Logic  AllPortsSameDT=off  OutDataTypeStr=boolean
  ForceRungInFalseRead : Subsystem  DisableCoverage=on  TreatAsAtomicUnit=on  mask{PLCLabelTag=_Force_RungIn_False, PLCBlockType=ForceRungInFalseRead}
      mask prompts: PLCLabelTag "Label Tag:"
      mask init:
      | block = gcb;
      | maskObj = Simulink.Mask.get(block);
      | maskObj.Display = sprintf('disp(''%s'');', PLCLabelTag);
      mask Help: web([docroot '/plccoder/ref/forcerunginfalseread' '.html']);
      mask DialogControl PLCBlockTitle Prompt: Force Rung-In False Read
      mask Display: disp('_Force_RungIn_False');
  NOT : Logic  Operator=NOT  IconShape=distinctive  AllPortsSameDT=off  OutDataTypeStr=boolean
  Out1 : Outport  VectorParamsAs1DForOutWhenUnconnected=off
  wires:
  AND/1 -> Out1/1
  In1/1 -> AND/2
  ForceRungInFalseRead/1(Out1) -> NOT/1
  NOT/1 -> AND/1

== system MIMO_FixedIO/PLC Controller Suite/__Logic/Task/Program/__Logic/OTE1/__CoreVarRead ==
  DataRead : DataStoreRead  DataStoreName=xxx_PLC_VAR_State1  IndexOptions=Index vector (dialog)  Indices=1  OutputSizes=1
  y : Outport  VectorParamsAs1DForOutWhenUnconnected=off
  wires:
  DataRead/1 -> y/1

== system MIMO_FixedIO/PLC Controller Suite/__Logic/Task/Program/__Logic/OTE2/BlockEnableRead ==
  __CoreLabelRead : Subsystem  Tag=CoreVarReadBlock  DisableCoverage=on  TreatAsAtomicUnit=on  mask{PLCBlockType=CoreLabelRead}
      mask init:
      | slplc.callbacks.initRoutineLabelRead(gcb);
      mask Help: web([docroot '/plccoder/ref/__corelabelread' '.html']);
      mask DialogControl PLCBlockTitle Prompt: Core Label Read
  Out1 : Outport  VectorParamsAs1DForOutWhenUnconnected=off
  wires:
  __CoreLabelRead/1(Out1) -> Out1/1

== system MIMO_FixedIO/PLC Controller Suite/__Logic/Task/Program/__Logic/OTE2/Instruction_Enable ==
  Rung-condition-in : Inport  OutDataTypeStr=BOOL
  Enable : EnablePort
  Initialize Function : Subsystem  TreatAsAtomicUnit=on
  NOT : Logic  Operator=NOT  IconShape=distinctive  AllPortsSameDT=off  OutDataTypeStr=boolean
  Rung-condition is false : Subsystem  Priority=12  DisableCoverage=on
  Rung-condition-in is true : Subsystem  Priority=12  DisableCoverage=on
  wires:
  NOT/1 -> Rung-condition is false/Enable
  Rung-condition-in/1 -> Rung-condition-in is true/Enable, NOT/1  "Rung-condition-in"

== system MIMO_FixedIO/PLC Controller Suite/__Logic/Task/Program/__Logic/OTE2/RungInOverride ==
  In1 : Inport
  AND : Logic  AllPortsSameDT=off  OutDataTypeStr=boolean
  ForceRungInFalseRead : Subsystem  DisableCoverage=on  TreatAsAtomicUnit=on  mask{PLCLabelTag=_Force_RungIn_False, PLCBlockType=ForceRungInFalseRead}
      mask prompts: PLCLabelTag "Label Tag:"
      mask init:
      | block = gcb;
      | maskObj = Simulink.Mask.get(block);
      | maskObj.Display = sprintf('disp(''%s'');', PLCLabelTag);
      mask Help: web([docroot '/plccoder/ref/forcerunginfalseread' '.html']);
      mask DialogControl PLCBlockTitle Prompt: Force Rung-In False Read
      mask Display: disp('_Force_RungIn_False');
  NOT : Logic  Operator=NOT  IconShape=distinctive  AllPortsSameDT=off  OutDataTypeStr=boolean
  Out1 : Outport  VectorParamsAs1DForOutWhenUnconnected=off
  wires:
  AND/1 -> Out1/1
  In1/1 -> AND/2
  ForceRungInFalseRead/1(Out1) -> NOT/1
  NOT/1 -> AND/1

== system MIMO_FixedIO/PLC Controller Suite/__Logic/Task/Program/__Logic/OTE2/__CoreVarRead ==
  DataRead : DataStoreRead  DataStoreName=xxx_PLC_VAR_M1  IndexOptions=Index vector (dialog)  Indices=1  OutputSizes=1
  y : Outport  VectorParamsAs1DForOutWhenUnconnected=off
  wires:
  DataRead/1 -> y/1

== system MIMO_FixedIO/PLC Controller Suite/__Logic/Task/Program/__Logic/OTE3/BlockEnableRead ==
  __CoreLabelRead : Subsystem  Tag=CoreVarReadBlock  DisableCoverage=on  TreatAsAtomicUnit=on  mask{PLCBlockType=CoreLabelRead}
      mask init:
      | slplc.callbacks.initRoutineLabelRead(gcb);
      mask Help: web([docroot '/plccoder/ref/__corelabelread' '.html']);
      mask DialogControl PLCBlockTitle Prompt: Core Label Read
  Out1 : Outport  VectorParamsAs1DForOutWhenUnconnected=off
  wires:
  __CoreLabelRead/1(Out1) -> Out1/1

== system MIMO_FixedIO/PLC Controller Suite/__Logic/Task/Program/__Logic/OTE3/Instruction_Enable ==
  Rung-condition-in : Inport  OutDataTypeStr=BOOL
  Enable : EnablePort
  Initialize Function : Subsystem  TreatAsAtomicUnit=on
  NOT : Logic  Operator=NOT  IconShape=distinctive  AllPortsSameDT=off  OutDataTypeStr=boolean
  Rung-condition is false : Subsystem  Priority=12  DisableCoverage=on
  Rung-condition-in is true : Subsystem  Priority=12  DisableCoverage=on
  wires:
  NOT/1 -> Rung-condition is false/Enable
  Rung-condition-in/1 -> Rung-condition-in is true/Enable, NOT/1  "Rung-condition-in"

== system MIMO_FixedIO/PLC Controller Suite/__Logic/Task/Program/__Logic/OTE3/RungInOverride ==
  In1 : Inport
  AND : Logic  AllPortsSameDT=off  OutDataTypeStr=boolean
  ForceRungInFalseRead : Subsystem  DisableCoverage=on  TreatAsAtomicUnit=on  mask{PLCLabelTag=_Force_RungIn_False, PLCBlockType=ForceRungInFalseRead}
      mask prompts: PLCLabelTag "Label Tag:"
      mask init:
      | block = gcb;
      | maskObj = Simulink.Mask.get(block);
      | maskObj.Display = sprintf('disp(''%s'');', PLCLabelTag);
      mask Help: web([docroot '/plccoder/ref/forcerunginfalseread' '.html']);
      mask DialogControl PLCBlockTitle Prompt: Force Rung-In False Read
      mask Display: disp('_Force_RungIn_False');
  NOT : Logic  Operator=NOT  IconShape=distinctive  AllPortsSameDT=off  OutDataTypeStr=boolean
  Out1 : Outport  VectorParamsAs1DForOutWhenUnconnected=off
  wires:
  AND/1 -> Out1/1
  In1/1 -> AND/2
  ForceRungInFalseRead/1(Out1) -> NOT/1
  NOT/1 -> AND/1

== system MIMO_FixedIO/PLC Controller Suite/__Logic/Task/Program/__Logic/OTE3/__CoreVarRead ==
  DataRead : DataStoreRead  DataStoreName=xxx_PLC_VAR_M2  IndexOptions=Index vector (dialog)  Indices=1  OutputSizes=1
  y : Outport  VectorParamsAs1DForOutWhenUnconnected=off
  wires:
  DataRead/1 -> y/1

== system MIMO_FixedIO/PLC Controller Suite/__Logic/Task/Program/__Logic/OTE4/BlockEnableRead ==
  __CoreLabelRead : Subsystem  Tag=CoreVarReadBlock  DisableCoverage=on  TreatAsAtomicUnit=on  mask{PLCBlockType=CoreLabelRead}
      mask init:
      | slplc.callbacks.initRoutineLabelRead(gcb);
      mask Help: web([docroot '/plccoder/ref/__corelabelread' '.html']);
      mask DialogControl PLCBlockTitle Prompt: Core Label Read
  Out1 : Outport  VectorParamsAs1DForOutWhenUnconnected=off
  wires:
  __CoreLabelRead/1(Out1) -> Out1/1

== system MIMO_FixedIO/PLC Controller Suite/__Logic/Task/Program/__Logic/OTE4/Instruction_Enable ==
  Rung-condition-in : Inport  OutDataTypeStr=BOOL
  Enable : EnablePort
  Initialize Function : Subsystem  TreatAsAtomicUnit=on
  NOT : Logic  Operator=NOT  IconShape=distinctive  AllPortsSameDT=off  OutDataTypeStr=boolean
  Rung-condition is false : Subsystem  Priority=12  DisableCoverage=on
  Rung-condition-in is true : Subsystem  Priority=12  DisableCoverage=on
  wires:
  NOT/1 -> Rung-condition is false/Enable
  Rung-condition-in/1 -> Rung-condition-in is true/Enable, NOT/1  "Rung-condition-in"

== system MIMO_FixedIO/PLC Controller Suite/__Logic/Task/Program/__Logic/OTE4/RungInOverride ==
  In1 : Inport
  AND : Logic  AllPortsSameDT=off  OutDataTypeStr=boolean
  ForceRungInFalseRead : Subsystem  DisableCoverage=on  TreatAsAtomicUnit=on  mask{PLCLabelTag=_Force_RungIn_False, PLCBlockType=ForceRungInFalseRead}
      mask prompts: PLCLabelTag "Label Tag:"
      mask init:
      | block = gcb;
      | maskObj = Simulink.Mask.get(block);
      | maskObj.Display = sprintf('disp(''%s'');', PLCLabelTag);
      mask Help: web([docroot '/plccoder/ref/forcerunginfalseread' '.html']);
      mask DialogControl PLCBlockTitle Prompt: Force Rung-In False Read
      mask Display: disp('_Force_RungIn_False');
  NOT : Logic  Operator=NOT  IconShape=distinctive  AllPortsSameDT=off  OutDataTypeStr=boolean
  Out1 : Outport  VectorParamsAs1DForOutWhenUnconnected=off
  wires:
  AND/1 -> Out1/1
  In1/1 -> AND/2
  ForceRungInFalseRead/1(Out1) -> NOT/1
  NOT/1 -> AND/1

== system MIMO_FixedIO/PLC Controller Suite/__Logic/Task/Program/__Logic/OTE4/__CoreVarRead ==
  DataRead : DataStoreRead  DataStoreName=xxx_PLC_VAR_State2  IndexOptions=Index vector (dialog)  Indices=1  OutputSizes=1
  y : Outport  VectorParamsAs1DForOutWhenUnconnected=off
  wires:
  DataRead/1 -> y/1

== system MIMO_FixedIO/PLC Controller Suite/__Logic/Task/Program/__Logic/XIC/BlockEnableRead ==
  __CoreLabelRead : Subsystem  Tag=CoreVarReadBlock  DisableCoverage=on  TreatAsAtomicUnit=on  mask{PLCBlockType=CoreLabelRead}
      mask init:
      | slplc.callbacks.initRoutineLabelRead(gcb);
      mask Help: web([docroot '/plccoder/ref/__corelabelread' '.html']);
      mask DialogControl PLCBlockTitle Prompt: Core Label Read
  Out1 : Outport  VectorParamsAs1DForOutWhenUnconnected=off
  wires:
  __CoreLabelRead/1(Out1) -> Out1/1

== system MIMO_FixedIO/PLC Controller Suite/__Logic/Task/Program/__Logic/XIC/Instruction_Enable ==
  Rung-condition-in : Inport  OutDataTypeStr=BOOL
  Enable : EnablePort
  Logical Operator : Logic  OutDataTypeStr=BOOL
  __CoreVarRead : Subsystem  Tag=CoreVarReadBlock  DisableCoverage=on  TreatAsAtomicUnit=on  mask{PLCBlockType=CoreVarRead}
      mask init:
      | slplc.callbacks.initCoreVariable(gcb, 'read');
      mask Help: web([docroot '/plccoder/ref/__corevarread' '.html']);
      mask DialogControl PLCBlockTitle Prompt: Core Variable Read
  Rung-condition-out : Outport  VectorParamsAs1DForOutWhenUnconnected=off
  wires:
  Rung-condition-in/1 -> Logical Operator/1  "Rung-condition-in"
  Logical Operator/1 -> Rung-condition-out/1  "Rung-condition-out"
  __CoreVarRead/1(y) -> Logical Operator/2  "DataBit"

== system MIMO_FixedIO/PLC Controller Suite/__Logic/Task/Program/__Logic/XIC/RungInOverride ==
  In1 : Inport
  AND : Logic  AllPortsSameDT=off  OutDataTypeStr=boolean
  ForceRungInFalseRead : Subsystem  DisableCoverage=on  TreatAsAtomicUnit=on  mask{PLCLabelTag=_Force_RungIn_False, PLCBlockType=ForceRungInFalseRead}
      mask prompts: PLCLabelTag "Label Tag:"
      mask init:
      | block = gcb;
      | maskObj = Simulink.Mask.get(block);
      | maskObj.Display = sprintf('disp(''%s'');', PLCLabelTag);
      mask Help: web([docroot '/plccoder/ref/forcerunginfalseread' '.html']);
      mask DialogControl PLCBlockTitle Prompt: Force Rung-In False Read
      mask Display: disp('_Force_RungIn_False');
  NOT : Logic  Operator=NOT  IconShape=distinctive  AllPortsSameDT=off  OutDataTypeStr=boolean
  Out1 : Outport  VectorParamsAs1DForOutWhenUnconnected=off
  wires:
  AND/1 -> Out1/1
  In1/1 -> AND/2
  ForceRungInFalseRead/1(Out1) -> NOT/1
  NOT/1 -> AND/1

== system MIMO_FixedIO/PLC Controller Suite/__Logic/Task/Program/__Logic/XIC/__CoreVarRead ==
  DataRead : DataStoreRead  DataStoreName=xxx_PLC_VAR_State0  IndexOptions=Index vector (dialog)  Indices=1  OutputSizes=1
  y : Outport  VectorParamsAs1DForOutWhenUnconnected=off
  wires:
  DataRead/1 -> y/1

== system MIMO_FixedIO/PLC Controller Suite/__Logic/Task/Program/__Logic/XIC1/BlockEnableRead ==
  __CoreLabelRead : Subsystem  Tag=CoreVarReadBlock  DisableCoverage=on  TreatAsAtomicUnit=on  mask{PLCBlockType=CoreLabelRead}
      mask init:
      | slplc.callbacks.initRoutineLabelRead(gcb);
      mask Help: web([docroot '/plccoder/ref/__corelabelread' '.html']);
      mask DialogControl PLCBlockTitle Prompt: Core Label Read
  Out1 : Outport  VectorParamsAs1DForOutWhenUnconnected=off
  wires:
  __CoreLabelRead/1(Out1) -> Out1/1

== system MIMO_FixedIO/PLC Controller Suite/__Logic/Task/Program/__Logic/XIC1/Instruction_Enable ==
  Rung-condition-in : Inport  OutDataTypeStr=BOOL
  Enable : EnablePort
  Logical Operator : Logic  OutDataTypeStr=BOOL
  __CoreVarRead : Subsystem  Tag=CoreVarReadBlock  DisableCoverage=on  TreatAsAtomicUnit=on  mask{PLCBlockType=CoreVarRead}
      mask init:
      | slplc.callbacks.initCoreVariable(gcb, 'read');
      mask Help: web([docroot '/plccoder/ref/__corevarread' '.html']);
      mask DialogControl PLCBlockTitle Prompt: Core Variable Read
  Rung-condition-out : Outport  VectorParamsAs1DForOutWhenUnconnected=off
  wires:
  Rung-condition-in/1 -> Logical Operator/1  "Rung-condition-in"
  Logical Operator/1 -> Rung-condition-out/1  "Rung-condition-out"
  __CoreVarRead/1(y) -> Logical Operator/2  "DataBit"

== system MIMO_FixedIO/PLC Controller Suite/__Logic/Task/Program/__Logic/XIC1/RungInOverride ==
  In1 : Inport
  AND : Logic  AllPortsSameDT=off  OutDataTypeStr=boolean
  ForceRungInFalseRead : Subsystem  DisableCoverage=on  TreatAsAtomicUnit=on  mask{PLCLabelTag=_Force_RungIn_False, PLCBlockType=ForceRungInFalseRead}
      mask prompts: PLCLabelTag "Label Tag:"
      mask init:
      | block = gcb;
      | maskObj = Simulink.Mask.get(block);
      | maskObj.Display = sprintf('disp(''%s'');', PLCLabelTag);
      mask Help: web([docroot '/plccoder/ref/forcerunginfalseread' '.html']);
      mask DialogControl PLCBlockTitle Prompt: Force Rung-In False Read
      mask Display: disp('_Force_RungIn_False');
  NOT : Logic  Operator=NOT  IconShape=distinctive  AllPortsSameDT=off  OutDataTypeStr=boolean
  Out1 : Outport  VectorParamsAs1DForOutWhenUnconnected=off
  wires:
  AND/1 -> Out1/1
  In1/1 -> AND/2
  ForceRungInFalseRead/1(Out1) -> NOT/1
  NOT/1 -> AND/1

== system MIMO_FixedIO/PLC Controller Suite/__Logic/Task/Program/__Logic/XIC1/__CoreVarRead ==
  DataRead : DataStoreRead  DataStoreName=xxx_PLC_VAR_B1  IndexOptions=Index vector (dialog)  Indices=1  OutputSizes=1
  y : Outport  VectorParamsAs1DForOutWhenUnconnected=off
  wires:
  DataRead/1 -> y/1

== system MIMO_FixedIO/PLC Controller Suite/__Logic/Task/Program/__Logic/XIC2/BlockEnableRead ==
  __CoreLabelRead : Subsystem  Tag=CoreVarReadBlock  DisableCoverage=on  TreatAsAtomicUnit=on  mask{PLCBlockType=CoreLabelRead}
      mask init:
      | slplc.callbacks.initRoutineLabelRead(gcb);
      mask Help: web([docroot '/plccoder/ref/__corelabelread' '.html']);
      mask DialogControl PLCBlockTitle Prompt: Core Label Read
  Out1 : Outport  VectorParamsAs1DForOutWhenUnconnected=off
  wires:
  __CoreLabelRead/1(Out1) -> Out1/1
